simulink model "IEEE9_BUS_with2VSC_VI"  (R2019b)
settings: Solver=ode23tb  StartTime=0.0  StopTime=Tend  RelTol=1e-3
values from neighbouring files (symbols this model uses):
  C_4 = 0.1670*C_b    (= 1.00487241952e-06)    [Basic_Model_Works.m]    (also in VSC_GridFroming_Thesis_Script.m; VSC_GridFroming_Thesis_Script_withSynchMach.m)
  C_6 = 0.2835*C_b    (= 1.70587623314e-06)    [Basic_Model_Works.m]    (also in VSC_GridFroming_Thesis_Script.m; VSC_GridFroming_Thesis_Script_withSynchMach.m)
  C_8 = 0.2275*C_b    (= 1.36891302659e-06)    [Basic_Model_Works.m]    (also in VSC_GridFroming_Thesis_Script.m; VSC_GridFroming_Thesis_Script_withSynchMach.m)
  C_dc = 0.008*(n)    (= 1.6)    [Basic_Model_Works.m]    (also in VSC_GridFroming_Thesis_Script.m; VSC_GridFroming_Thesis_Script_withSynchMach.m)
  C_f = C_f_pu*C1_b    (= 0.0318309886184)    [Basic_Model_Works.m]    (also in VSC_GridFroming_Thesis_Script.m = 0.06; VSC_GridFroming_Thesis_Script_withSynchMach.m)
  droop_percentage = 1    [Basic_Model_Works.m]    (also in VSC_GridFroming_Thesis_Script.m; VSC_GridFroming_Thesis_Script_withSynchMach.m = 5)
  f_b = 50    [Basic_Model_Works.m]    (also in VSC_GridFroming_Thesis_Script.m; VSC_GridFroming_Thesis_Script_withSynchMach.m)
  I_b_LV = S_b/(sqrt(3)*V1_rms)    [Basic_Model_Works.m]    (also in VSC_GridFroming_Thesis_Script.m; VSC_GridFroming_Thesis_Script_withSynchMach.m)
  i_ll = -1.15*(S_b/Vdc_n)-i_loss_dc    [Basic_Model_Works.m]    (also in VSC_GridFroming_Thesis_Script.m; VSC_GridFroming_Thesis_Script_withSynchMach.m)
  I_threshold = I_thresh    (= 1)    [Basic_Model_Works.m]
  i_ul = 1.15*(S_b/Vdc_n)+i_loss_dc    [Basic_Model_Works.m]    (also in VSC_GridFroming_Thesis_Script.m; VSC_GridFroming_Thesis_Script_withSynchMach.m)
  k_dc = eta_1/(Vdc_n*m_p)    [Basic_Model_Works.m]    (also in VSC_GridFroming_Thesis_Script.m; VSC_GridFroming_Thesis_Script_withSynchMach.m)
  K_p = (1/Vdc_n)    [Basic_Model_Works.m]    (also in VSC_GridFroming_Thesis_Script.m; VSC_GridFroming_Thesis_Script_withSynchMach.m)
  K_r = 1/R_dc    [Basic_Model_Works.m]    (also in VSC_GridFroming_Thesis_Script.m; VSC_GridFroming_Thesis_Script_withSynchMach.m)
  Kff_i = 1    [Basic_Model_Works.m]    (also in VSC_GridFroming_Thesis_Script.m; VSC_GridFroming_Thesis_Script_withSynchMach.m)
  Kff_v = 1    [Basic_Model_Works.m]    (also in VSC_GridFroming_Thesis_Script.m; VSC_GridFroming_Thesis_Script_withSynchMach.m)
  Ki_i = (1/n)*1.19    (= 0.00595)    [Basic_Model_Works.m]    (also in VSC_GridFroming_Thesis_Script.m; VSC_GridFroming_Thesis_Script_withSynchMach.m)
  Ki_v = (n)*1.16    (= 232)    [Basic_Model_Works.m]    (also in VSC_GridFroming_Thesis_Script.m = 232.2044; VSC_GridFroming_Thesis_Script_withSynchMach.m = 232.2044)
  ki_v_ac = 10    [Basic_Model_Works.m]    (also in VSC_GridFroming_Thesis_Script.m = 0.5; VSC_GridFroming_Thesis_Script_withSynchMach.m)
  Kp_i = 0.73    [Basic_Model_Works.m]    (also in VSC_GridFroming_Thesis_Script.m = 0.738891; VSC_GridFroming_Thesis_Script_withSynchMach.m = 0.738891)
  Kp_v = 0.52    [Basic_Model_Works.m]    (also in VSC_GridFroming_Thesis_Script.m; VSC_GridFroming_Thesis_Script_withSynchMach.m)
  kp_v_ac = 0.05    [Basic_Model_Works.m]    (also in VSC_GridFroming_Thesis_Script.m = 0.001; VSC_GridFroming_Thesis_Script_withSynchMach.m)
  L1_pu = 1*0.0186/m    (= 0.000186)    [Basic_Model_Works.m]    (also in VSC_GridFroming_Thesis_Script.m; VSC_GridFroming_Thesis_Script_withSynchMach.m)
  L2_mh = 0.08    [Basic_Model_Works.m]    (also in VSC_GridFroming_Thesis_Script_withSynchMach.m)
  L_45 = L_lines(2)    [Basic_Model_Works.m]    (also in VSC_GridFroming_Thesis_Script.m; VSC_GridFroming_Thesis_Script_withSynchMach.m)
  L_56 = L_lines(3)    [Basic_Model_Works.m]    (also in VSC_GridFroming_Thesis_Script.m; VSC_GridFroming_Thesis_Script_withSynchMach.m)
  L_67 = L_lines(5)    [Basic_Model_Works.m]    (also in VSC_GridFroming_Thesis_Script.m; VSC_GridFroming_Thesis_Script_withSynchMach.m)
  L_78 = L_lines(6)    [Basic_Model_Works.m]    (also in VSC_GridFroming_Thesis_Script.m; VSC_GridFroming_Thesis_Script_withSynchMach.m)
  L_89 = L_lines(8)    [Basic_Model_Works.m]    (also in VSC_GridFroming_Thesis_Script.m; VSC_GridFroming_Thesis_Script_withSynchMach.m)
  L_94 = L_lines(9)    [Basic_Model_Works.m]    (also in VSC_GridFroming_Thesis_Script.m; VSC_GridFroming_Thesis_Script_withSynchMach.m)
  L_f = L_f_pu*L1_b    (= 4.77464829276e-06)    [Basic_Model_Works.m]    (also in VSC_GridFroming_Thesis_Script.m = 1e-06; VSC_GridFroming_Thesis_Script_withSynchMach.m)
  L_v = L_v_pu*L1_b    (= 9.54929658551e-06)    [Basic_Model_Works.m]    (also in VSC_GridFroming_Thesis_Script.m; VSC_GridFroming_Thesis_Script_withSynchMach.m = 1.59154943092e-07)
  load_step = S_b*load_change    (= 75000000)    [VSC_GridFroming_Thesis_Script.m]    (also in VSC_GridFroming_Thesis_Script_withSynchMach.m = 50000000)
  m_p = (50*(1.025)-  50*(0.975))/(n*VSC_Pn)    (= 1.25e-08)    [Basic_Model_Works.m]    (also in VSC_GridFroming_Thesis_Script.m = 3.14159265359e-08; VSC_GridFroming_Thesis_Script_withSynchMach.m)
  n = 200    [Basic_Model_Works.m]    (also in VSC_GridFroming_Thesis_Script.m; VSC_GridFroming_Thesis_Script_withSynchMach.m)
  Pn = 210* 1e6    (= 210000000)    [Basic_Model_Works.m]    (also in VSC_GridFroming_Thesis_Script_withSynchMach.m)
  ps = 0.67*Ptot_Load/n_gen    (= 0.5025)    [Basic_Model_Works.m]    (also in VSC_GridFroming_Thesis_Script.m = 0.75; VSC_GridFroming_Thesis_Script_withSynchMach.m = 0.65)
  R1_pu = 1*0.00734/m    (= 7.34e-05)    [Basic_Model_Works.m]    (also in VSC_GridFroming_Thesis_Script.m; VSC_GridFroming_Thesis_Script_withSynchMach.m)
  R2_mh = 0.0027    [Basic_Model_Works.m]    (also in VSC_GridFroming_Thesis_Script_withSynchMach.m)
  R_45 = R_lines(2)    [Basic_Model_Works.m]    (also in VSC_GridFroming_Thesis_Script.m; VSC_GridFroming_Thesis_Script_withSynchMach.m)
  R_56 = R_lines(3)    [Basic_Model_Works.m]    (also in VSC_GridFroming_Thesis_Script.m; VSC_GridFroming_Thesis_Script_withSynchMach.m)
  R_67 = R_lines(5)    [Basic_Model_Works.m]    (also in VSC_GridFroming_Thesis_Script.m; VSC_GridFroming_Thesis_Script_withSynchMach.m)
  R_78 = R_lines(6)    [Basic_Model_Works.m]    (also in VSC_GridFroming_Thesis_Script.m; VSC_GridFroming_Thesis_Script_withSynchMach.m)
  R_89 = R_lines(8)    [Basic_Model_Works.m]    (also in VSC_GridFroming_Thesis_Script.m; VSC_GridFroming_Thesis_Script_withSynchMach.m)
  R_94 = R_lines(9)    [Basic_Model_Works.m]    (also in VSC_GridFroming_Thesis_Script.m; VSC_GridFroming_Thesis_Script_withSynchMach.m)
  R_dc = (Vdc_n/(0.05*(S_b)/Vdc_n))    [Basic_Model_Works.m]    (also in VSC_GridFroming_Thesis_Script.m; VSC_GridFroming_Thesis_Script_withSynchMach.m)
  R_f = R_f_pu*Z1_b    (= 5e-05)    [Basic_Model_Works.m]    (also in VSC_GridFroming_Thesis_Script.m = 5e-06; VSC_GridFroming_Thesis_Script_withSynchMach.m)
  R_v = R_v_pu*Z1_b    (= 0.002)    [Basic_Model_Works.m]    (also in VSC_GridFroming_Thesis_Script.m = 0.001; VSC_GridFroming_Thesis_Script_withSynchMach.m = 1e-05)
  S_b = 100*(10^6)    (= 100000000)    [Basic_Model_Works.m]    (also in VSC_GridFroming_Thesis_Script.m; VSC_GridFroming_Thesis_Script_withSynchMach.m)
  T1sc_off = 13.15    [Basic_Model_Works.m]
  T1sc_on = 13    [Basic_Model_Works.m]
  T3sc_off = 30.15    [Basic_Model_Works.m]
  T3sc_on = 30    [Basic_Model_Works.m]
  T_conn = 13    [Basic_Model_Works.m]
  T_discon = 32    [Basic_Model_Works.m]
  T_en = T_conn-0.5    (= 12.5)    [Basic_Model_Works.m]    (also in VSC_GridFroming_Thesis_Script.m = 19.5; VSC_GridFroming_Thesis_Script_withSynchMach.m = 11.5)
  T_loss = Tend    (= 40)    [VSC_GridFroming_Thesis_Script.m]    (also in VSC_GridFroming_Thesis_Script_withSynchMach.m = 35)
  T_s = 1e-4    (= 0.0001)    [Basic_Model_Works.m]    (also in VSC_GridFroming_Thesis_Script.m; VSC_GridFroming_Thesis_Script_withSynchMach.m)
  tau_dc = 0.05    [Basic_Model_Works.m]    (also in VSC_GridFroming_Thesis_Script.m; VSC_GridFroming_Thesis_Script_withSynchMach.m)
  tau_g = 0.25    [Basic_Model_Works.m]    (also in VSC_GridFroming_Thesis_Script.m = 5; VSC_GridFroming_Thesis_Script_withSynchMach.m = 5)
  Tsc_off = 21.15    [Basic_Model_Works.m]    (also in VSC_GridFroming_Thesis_Script_withSynchMach.m = 20.25)
  Tsc_on = 21    [Basic_Model_Works.m]    (also in VSC_GridFroming_Thesis_Script_withSynchMach.m = 20)
  V = 230*(10^3)    (= 230000)    [Basic_Model_Works.m]    (also in VSC_GridFroming_Thesis_Script.m; VSC_GridFroming_Thesis_Script_withSynchMach.m)
  V1_rms = 1000    [Basic_Model_Works.m]    (also in VSC_GridFroming_Thesis_Script.m; VSC_GridFroming_Thesis_Script_withSynchMach.m)
  V2_rms = 13800    [Basic_Model_Works.m]    (also in VSC_GridFroming_Thesis_Script.m; VSC_GridFroming_Thesis_Script_withSynchMach.m)
  V_m = sqrt(2/3)*V1_rms    [Basic_Model_Works.m]    (also in VSC_GridFroming_Thesis_Script.m; VSC_GridFroming_Thesis_Script_withSynchMach.m)
  Vdc_n = 3*V_m    [Basic_Model_Works.m]    (also in VSC_GridFroming_Thesis_Script.m; VSC_GridFroming_Thesis_Script_withSynchMach.m)
  w_c = w_ref/4.95    (= 63.4665182543)    [Basic_Model_Works.m]    (also in VSC_GridFroming_Thesis_Script_withSynchMach.m)
  w_f = 7.5    [Basic_Model_Works.m]    (also in VSC_GridFroming_Thesis_Script.m = 31.4159265359; VSC_GridFroming_Thesis_Script_withSynchMach.m)
  w_ref = 2*pi*f_b    (= 314.159265359)    [Basic_Model_Works.m]    (also in VSC_GridFroming_Thesis_Script.m; VSC_GridFroming_Thesis_Script_withSynchMach.m)
undefined symbols (not defined in the file or in its folder): D1, Delta, i_dc
libraries: powerlib x112, powerlib_meascontrol x40, cstblocks x5, simulink x4, sps_avr x1
(part 3 of 3)

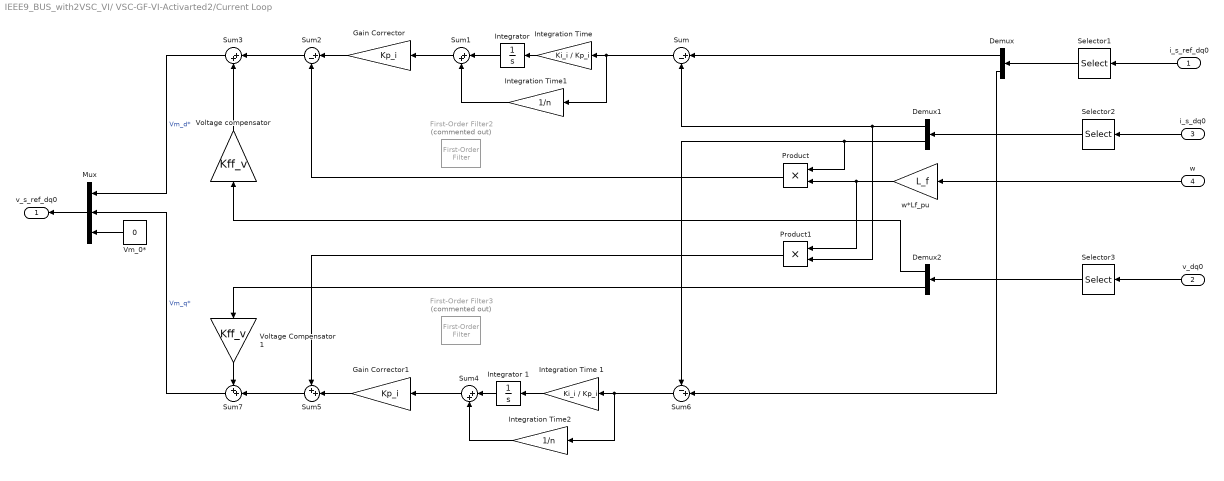
== system IEEE9_BUS_with2VSC_VI/ VSC-GF-VI-Activarted2/Current Loop ==
  i_s_ref_dq0 : Inport
  v_dq0 : Inport  Port=2
  i_s_dq0 : Inport  Port=3
  w : Inport  Port=4
  Demux : Demux  Outputs=2
  Demux1 : Demux  Outputs=2
  Demux2 : Demux  Outputs=2
  First-Order Filter2 : powerlib_meascontrol/Filters/First-Order Filter  Commented=on  FilterType=Lowpass  Tc=25e-3  Ts=0  Initialize=on  Vac_Init=[0, 0, 50]  Vdc_Init=1  PlotResponse=off  FreqRange="[0,  200,  1]"
      settings: SourceProductName=Simscape Electrical
  First-Order Filter3 : powerlib_meascontrol/Filters/First-Order Filter  Commented=on  FilterType=Lowpass  Tc=25e-3  Ts=0  Initialize=on  Vac_Init=[0, 0, 50]  Vdc_Init=0  PlotResponse=off  FreqRange="[0,  200,  1]"
      settings: SourceProductName=Simscape Electrical
  Gain Corrector : Gain  Gain=Kp_i
  Gain Corrector1 : Gain  Gain=Kp_i
  Integration Time : Gain  Gain=Ki_i / Kp_i
  Integration Time 1 : Gain  Gain=Ki_i / Kp_i
  Integration Time1 : Gain  Gain=1/n
  Integration Time2 : Gain  Gain=1/n
  Integrator : Integrator  InitialCondition=0.0001
  Integrator 1 : Integrator
  Mux : Mux  Inputs=3
  Product : Product  RndMeth=Zero
  Product1 : Product  RndMeth=Zero
  Selector1 : Selector  InputPortWidth=3  IndexOptions=Index vector (dialog)  Indices=[1 2]  OutputSizes=1
  Selector2 : Selector  InputPortWidth=3  IndexOptions=Index vector (dialog)  Indices=[1 2]  OutputSizes=1
  Selector3 : Selector  InputPortWidth=3  IndexOptions=Index vector (dialog)  Indices=[1 2]  OutputSizes=1
  Sum : Sum  Inputs=|+-
  Sum1 : Sum  Inputs=|++
  Sum2 : Sum  Inputs=|+-
  Sum3 : Sum  Inputs=|++
  Sum4 : Sum  Inputs=|++
  Sum5 : Sum  Inputs=++|
  Sum6 : Sum  Inputs=-+|
  Sum7 : Sum  Inputs=++|
  Vm_0* : Constant  Value=0
  Voltage Compensator 1 : Gain  Gain=Kff_v
  Voltage compensator : Gain  Gain=Kff_v
  w*Lf_pu : Gain  Gain=L_f
  v_s_ref_dq0 : Outport  VectorParamsAs1DForOutWhenUnconnected=off
  wires:
  Sum/1 -> Integration Time/1, Integration Time1/1
  Integration Time 1/1 -> Integrator 1/1
  Integration Time/1 -> Integrator/1
  Sum5/1 -> Sum7/2
  Sum6/1 -> Integration Time 1/1, Integration Time2/1
  Demux/1 -> Sum/1
  Sum3/1 -> Mux/1  "Vm_d*"
  Sum7/1 -> Mux/2  "Vm_q*"
  Demux2/2 -> Voltage Compensator 1/1
  Voltage Compensator 1/1 -> Sum7/1
  Product/1 -> Sum2/2
  w*Lf_pu/1 -> Product1/1, Product/2
  i_s_ref_dq0/1 -> Selector1/1
  v_dq0/1 -> Selector3/1
  Integrator 1/1 -> Sum4/1
  Voltage compensator/1 -> Sum3/2
  Sum1/1 -> Gain Corrector/1
  Sum2/1 -> Sum3/1
  Sum4/1 -> Gain Corrector1/1
  Demux/2 -> Sum6/2
  Selector1/1 -> Demux/1
  Gain Corrector/1 -> Sum2/1
  w/1 -> w*Lf_pu/1
  Mux/1 -> v_s_ref_dq0/1
  Selector2/1 -> Demux1/1
  i_s_dq0/1 -> Selector2/1
  Selector3/1 -> Demux2/1
  Demux1/2 -> Product/1, Sum6/1
  Vm_0*/1 -> Mux/3
  Integrator/1 -> Sum1/1
  Demux1/1 -> Product1/2, Sum/2
  Demux2/1 -> Voltage compensator/1
  Product1/1 -> Sum5/1
  Gain Corrector1/1 -> Sum5/2
  Integration Time1/1 -> Sum1/2
  Integration Time2/1 -> Sum4/2

== system IEEE9_BUS_with2VSC_VI/ VSC-GF-VI-Activarted2/Droop Control ==
  w_b : Inport
  p_m : Inport  Port=2
  p_set : Inport  Port=3
  v_m : Inport  Port=4
  V_abc : Inport  Port=5
  Demux : Demux  Outputs=3
  Gain20 : Gain  Gain=m_p
  Integrator3 : Integrator
  Mux4 : Mux  Inputs=3
  PID Controller : simulink/Continuous/PID Controller  Controller=PID  Form=Parallel  TimeDomain=Continuous-time  SampleTime=-1  IntegratorMethod=Forward Euler  FilterMethod=Forward Euler  ControllerParametersSource=internal  P=kp_v_ac  I=ki_v_ac  D=0  UseFilter=on  N=100  TunerSelectOption=Transfer Function Based (PID Tuner App)  InitialConditionSource=internal  InitialConditionForIntegrator=0  InitialConditionForFilter=0  DifferentiatorICPrevScaledInput=0  ExternalReset=none  TrackingMode=off  Kt=1  LimitOutput=off  UpperSaturationLimit=inf  LowerSaturationLimit=-inf  LinearizeAsGain=on  AntiWindupMode=none  Kb=1  POutMin=[]  POutMax=[]  IOutMin=[]  IOutMax=[]  DOutMin=[]  DOutMax=[]  NOutMin=[]  NOutMax=[]  SumOutMin=[]  SumOutMax=[]  SaturationOutMin=[]  SaturationOutMax=[]  PParamMin=[]  PParamMax=[]  IParamMin=[]  IParamMax=[]  DParamMin=[]  DParamMax=[]  NParamMin=[]  NParamMax=[]  KbParamMin=[]  KbParamMax=[]  KtParamMin=[]  KtParamMax=[]  KbOutMin=[]  KbOutMax=[]  KtOutMin=[]  KtOutMax=[]  IntegratorOutMin=[]  IntegratorOutMax=[]  FilterOutMin=[]  FilterOutMax=[]  SumI1OutMin=[]  SumI1OutMax=[]  SumI2OutMin=[]  SumI2OutMax=[]  SumI3OutMin=[]  SumI3OutMax=[]  SumI4OutMin=[]  SumI4OutMax=[]  SumDOutMin=[]  SumDOutMax=[]  DifferentiatorOutMin=[]  DifferentiatorOutMax=[]  FilterDiffOutCoefMin=[]  FilterDiffOutCoefMax=[]  ReciprocalOutMin=[]  ReciprocalOutMax=[]  SumDenOutMin=[]  SumDenOutMax=[]  SumNumOutMin=[]  SumNumOutMax=[]  DivideOutMin=[]  DivideOutMax=[]  IntegratorContinuousStateAttributes=''  IntegratorStateMustResolveToSignalObject=off  IntegratorRTWStateStorageClass=Auto  FilterContinuousStateAttributes=''  FilterStateMustResolveToSignalObject=off  FilterRTWStateStorageClass=Auto  ParallelPVariant=InternalParameters  IdealPVariant=Disabled  IVariant=InternalParameters  DVariant=InternalParameters  IntegratorVariant=Continuous  SatVariant=Disabled  AWVariant=Passthrough  PCopyVariant=Disabled  TRVariant=Disabled  FdbkBlocksVariant=Forward  IdealPFdbkVariant=Disabled  SatFdbkVariant=Disabled  DerivativeFilterVariant=ContFilter  NVariant=InternalParameters  NCopyVariant=Disabled  FilterICVariant=InternalICsFilter  IntegratorICVariant=InternalICs  ExternalResetVariant=Disabled  TRSumVariant=Passthrough  SumFdbkVariant=Disabled  SumVariant=Sum_PID
  Sum1 : Sum  Inputs=-+|
  Sum7 : Sum  Inputs=|-+
  Sum8 : Sum  Inputs=++|
  Terminator : Terminator
  Terminator1 : Terminator
  Transfer Fcn1 : TransferFcn  Numerator=[w_f]  Denominator=[1 w_f]
  Transfer Fcn2 : TransferFcn  Numerator=[w_c]  Denominator=[1 w_c]
  abc to dq1 : powerlib_meascontrol/Transformations/abc to dq0  Alignment=90 degrees behind phase A axis
      settings: SourceProductName=Simscape Electrical
  q0 : Constant  Value=0
  w_ref : Outport  VectorParamsAs1DForOutWhenUnconnected=off
  theta_ref : Outport  Port=2  VectorParamsAs1DForOutWhenUnconnected=off
  v_ref_dq0 : Outport  Port=3  VectorParamsAs1DForOutWhenUnconnected=off
  wires:
  q0/1 -> Mux4/3, Mux4/2
  Sum8/1 -> Integrator3/1, w_ref/1
  p_set/1 -> Sum7/2
  w_b/1 -> Sum8/1
  Integrator3/1 -> theta_ref/1
  p_m/1 -> Transfer Fcn1/1
  Sum7/1 -> Gain20/1
  Transfer Fcn1/1 -> Sum7/1
  Gain20/1 -> Transfer Fcn2/1
  Transfer Fcn2/1 -> Sum8/2
  abc to dq1/1 -> Demux/1
  Demux/2 -> Terminator/1
  Demux/3 -> Terminator1/1
  v_m/1 -> Mux4/1
  Mux4/1 -> v_ref_dq0/1

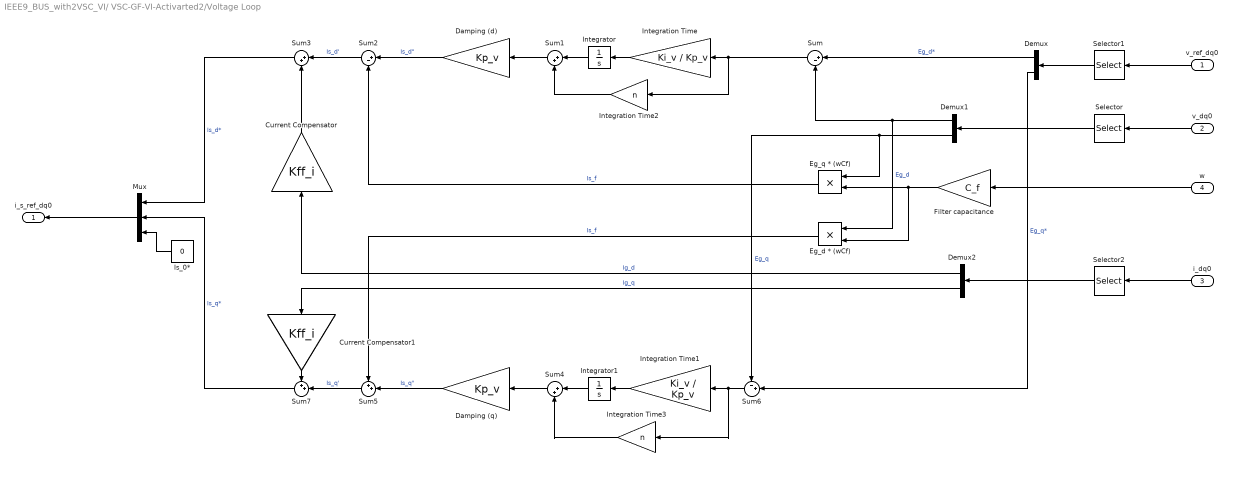
== system IEEE9_BUS_with2VSC_VI/ VSC-GF-VI-Activarted2/Voltage Loop ==
  v_ref_dq0 : Inport
  v_dq0 : Inport  Port=2
  i_dq0 : Inport  Port=3
  w : Inport  Port=4
  Current Compensator : Gain  Gain=Kff_i
  Current Compensator1 : Gain  Gain=Kff_i
  Damping (d) : Gain  Gain=Kp_v
  Damping (q) : Gain  Gain=Kp_v
  Demux : Demux  Outputs=2
  Demux1 : Demux  Outputs=2
  Demux2 : Demux  Outputs=2
  Eg_d * (wCf) : Product  RndMeth=Zero
  "Eg_q * (wCf) " : Product  RndMeth=Zero
  Filter capacitance : Gain  Gain=C_f
  Integration Time : Gain  Gain=Ki_v / Kp_v
  Integration Time1 : Gain  Gain=Ki_v / Kp_v
  Integration Time2 : Gain  Gain=n
  Integration Time3 : Gain  Gain=n
  Integrator : Integrator
  Integrator1 : Integrator
  Is_0* : Constant  Value=0
  Mux : Mux  Inputs=3
  Selector : Selector  InputPortWidth=3  IndexOptions=Index vector (dialog)  Indices=[1 2]  OutputSizes=1
  Selector1 : Selector  InputPortWidth=3  IndexOptions=Index vector (dialog)  Indices=[1 2]  OutputSizes=1
  Selector2 : Selector  InputPortWidth=3  IndexOptions=Index vector (dialog)  Indices=[1 2]  OutputSizes=1
  Sum : Sum  Inputs=|+-
  Sum1 : Sum  Inputs=|++
  Sum2 : Sum  Inputs=|+-
  Sum3 : Sum  Inputs=|++
  Sum4 : Sum  Inputs=|++
  Sum5 : Sum  Inputs=++|
  Sum6 : Sum  Inputs=-+|
  Sum7 : Sum  Inputs=++|
  i_s_ref_dq0 : Outport  VectorParamsAs1DForOutWhenUnconnected=off
  wires:
  Is_0*/1 -> Mux/3
  w/1 -> Filter capacitance/1
  Integration Time1/1 -> Integrator1/1
  Integrator1/1 -> Sum4/1
  Demux/2 -> Sum6/2  "Eg_q*"
  v_ref_dq0/1 -> Selector1/1
  Eg_d * (wCf)/1 -> Sum5/1  "Is_f"
  Sum7/1 -> Mux/2  "Is_q*"
  Demux2/2 -> Current Compensator1/1  "Ig_q"
  Demux/1 -> Sum/1  "Eg_d*"
  Sum6/1 -> Integration Time3/1, Integration Time1/1
  Demux2/1 -> Current Compensator/1  "Ig_d"
  Sum2/1 -> Sum3/1  "Is_d'"
  Current Compensator/1 -> Sum3/2
  Demux1/1 -> Eg_d * (wCf)/1, Sum/2  "Eg_d"
  Current Compensator1/1 -> Sum7/1
  "Eg_q * (wCf) "/1 -> Sum2/2  "Is_f"
  Demux1/2 -> "Eg_q * (wCf) "/1, Sum6/1  "Eg_q"
  Filter capacitance/1 -> "Eg_q * (wCf) "/2, Eg_d * (wCf)/2
  Damping (d)/1 -> Sum2/1  "Is_d\""
  i_dq0/1 -> Selector2/1
  Sum5/1 -> Sum7/2  "Is_q'"
  Sum1/1 -> Damping (d)/1
  Integrator/1 -> Sum1/1
  Integration Time/1 -> Integrator/1
  Sum4/1 -> Damping (q)/1
  Sum3/1 -> Mux/1  "Is_d*"
  v_dq0/1 -> Selector/1
  Damping (q)/1 -> Sum5/2  "Is_q\""
  Selector/1 -> Demux1/1
  Selector1/1 -> Demux/1
  Selector2/1 -> Demux2/1
  Mux/1 -> i_s_ref_dq0/1
  Sum/1 -> Integration Time/1, Integration Time2/1
  Integration Time2/1 -> Sum1/2
  Integration Time3/1 -> Sum4/2

== system IEEE9_BUS_with2VSC_VI/Synchronous Machine/Subsystem2 ==
  P_ref : Inport
  speed_ref : Inport  Port=2
  speed : Inport  Port=3
  1/droop : Gain  Gain=1/((droop_percentage/100))
  Delta load setpoint : Sum  Inputs=+-|
  Delta speed : Sum  Inputs=-+|
  throttle : Outport  VectorParamsAs1DForOutWhenUnconnected=off
  wires:
  speed/1 -> Delta speed/2
  1/droop/1 -> Delta load setpoint/2
  Delta speed/1 -> 1/droop/1
  speed_ref/1 -> Delta speed/1
  P_ref/1 -> Delta load setpoint/1
  Delta load setpoint/1 -> throttle/1

== system IEEE9_BUS_with2VSC_VI/VSC-GF-VI2/ Virtual Impedance ==
  "V_ref_P-w " : Inport
  I_dq0 : Inport  Port=2
  w : Inport  Port=3
  Constant : Constant  Value=0
  Demux4 : Demux  Outputs=2
  "Io_d * (w*Lv) " : Product  RndMeth=Zero
  "Io_q * (w*Lv) " : Product  RndMeth=Zero
  Mux : Mux  Inputs=3
  Selector : Selector  InputPortWidth=3  IndexOptions=Index vector (dialog)  Indices=[1 2]  OutputSizes=1
  Sum : Sum  Inputs=|+-
  Sum4 : Sum  Inputs=|++
  Sum5 : Sum  Inputs=-+|
  Sum6 : Sum  Inputs=-+|
  V_ref_0 : Constant  Value=0
  Virtual indutance : Gain  Gain=L_v
  Virtual resistance : Gain  Gain=R_v
  "Virtual resistance2 " : Gain  Gain=R_v
  V_ref_dq0_VI : Outport
  wires:
  "Io_d * (w*Lv) "/1 -> Sum5/1  "Io_d * (w*Lv)"
  Sum4/1 -> Mux/1
  Virtual indutance/1 -> "Io_q * (w*Lv) "/2, "Io_d * (w*Lv) "/2
  Sum/1 -> Sum4/1
  I_dq0/1 -> Selector/1
  w/1 -> Virtual indutance/1
  Virtual resistance/1 -> Sum/2
  "Virtual resistance2 "/1 -> Sum6/1
  Sum5/1 -> Mux/2
  Selector/1 -> Demux4/1
  Sum6/1 -> Sum5/2
  V_ref_0/1 -> Mux/3
  Demux4/1 -> "Io_d * (w*Lv) "/1, Virtual resistance/1  "Io_d"
  "V_ref_P-w "/1 -> Sum/1  "|v_ref|"
  Constant/1 -> Sum6/2
  "Io_q * (w*Lv) "/1 -> Sum4/2  "Io_q * (w*Lv)"
  Demux4/2 -> "Virtual resistance2 "/1, "Io_q * (w*Lv) "/1  "Io_q"
  Mux/1 -> V_ref_dq0_VI/1

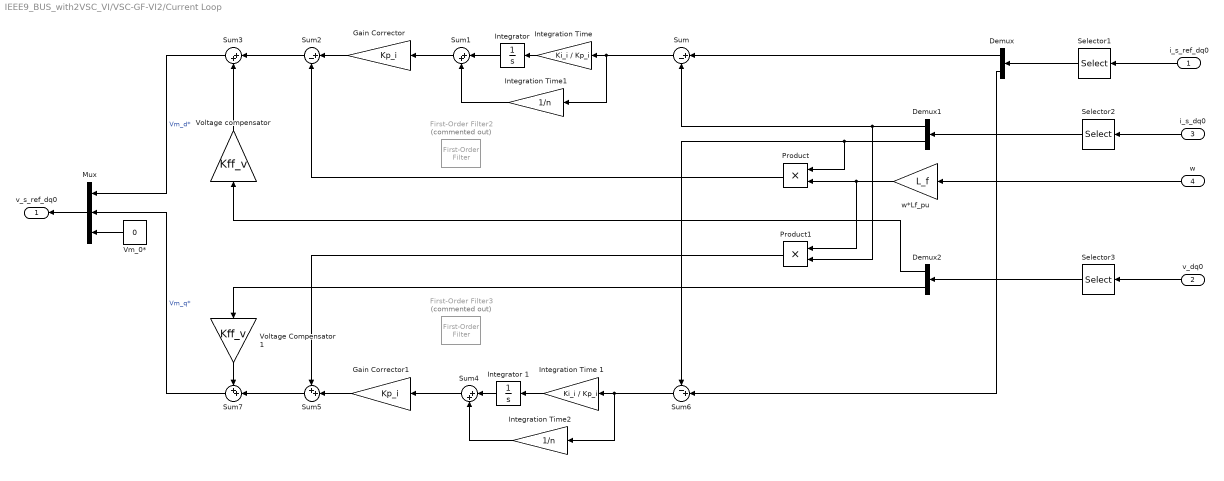
== system IEEE9_BUS_with2VSC_VI/VSC-GF-VI2/Current Loop ==
  i_s_ref_dq0 : Inport
  v_dq0 : Inport  Port=2
  i_s_dq0 : Inport  Port=3
  w : Inport  Port=4
  Demux : Demux  Outputs=2
  Demux1 : Demux  Outputs=2
  Demux2 : Demux  Outputs=2
  First-Order Filter2 : powerlib_meascontrol/Filters/First-Order Filter  Commented=on  FilterType=Lowpass  Tc=25e-3  Ts=0  Initialize=on  Vac_Init=[0, 0, 50]  Vdc_Init=1  PlotResponse=off  FreqRange="[0,  200,  1]"
      settings: SourceProductName=Simscape Electrical
  First-Order Filter3 : powerlib_meascontrol/Filters/First-Order Filter  Commented=on  FilterType=Lowpass  Tc=25e-3  Ts=0  Initialize=on  Vac_Init=[0, 0, 50]  Vdc_Init=0  PlotResponse=off  FreqRange="[0,  200,  1]"
      settings: SourceProductName=Simscape Electrical
  Gain Corrector : Gain  Gain=Kp_i
  Gain Corrector1 : Gain  Gain=Kp_i
  Integration Time : Gain  Gain=Ki_i / Kp_i
  Integration Time 1 : Gain  Gain=Ki_i / Kp_i
  Integration Time1 : Gain  Gain=1/n
  Integration Time2 : Gain  Gain=1/n
  Integrator : Integrator  InitialCondition=0.0001
  Integrator 1 : Integrator
  Mux : Mux  Inputs=3
  Product : Product  RndMeth=Zero
  Product1 : Product  RndMeth=Zero
  Selector1 : Selector  InputPortWidth=3  IndexOptions=Index vector (dialog)  Indices=[1 2]  OutputSizes=1
  Selector2 : Selector  InputPortWidth=3  IndexOptions=Index vector (dialog)  Indices=[1 2]  OutputSizes=1
  Selector3 : Selector  InputPortWidth=3  IndexOptions=Index vector (dialog)  Indices=[1 2]  OutputSizes=1
  Sum : Sum  Inputs=|+-
  Sum1 : Sum  Inputs=|++
  Sum2 : Sum  Inputs=|+-
  Sum3 : Sum  Inputs=|++
  Sum4 : Sum  Inputs=|++
  Sum5 : Sum  Inputs=++|
  Sum6 : Sum  Inputs=-+|
  Sum7 : Sum  Inputs=++|
  Vm_0* : Constant  Value=0
  Voltage Compensator 1 : Gain  Gain=Kff_v
  Voltage compensator : Gain  Gain=Kff_v
  w*Lf_pu : Gain  Gain=L_f
  v_s_ref_dq0 : Outport  VectorParamsAs1DForOutWhenUnconnected=off
  wires:
  Sum/1 -> Integration Time/1, Integration Time1/1
  Integration Time 1/1 -> Integrator 1/1
  Integration Time/1 -> Integrator/1
  Sum5/1 -> Sum7/2
  Sum6/1 -> Integration Time 1/1, Integration Time2/1
  Demux/1 -> Sum/1
  Sum3/1 -> Mux/1  "Vm_d*"
  Sum7/1 -> Mux/2  "Vm_q*"
  Demux2/2 -> Voltage Compensator 1/1
  Voltage Compensator 1/1 -> Sum7/1
  Product/1 -> Sum2/2
  w*Lf_pu/1 -> Product1/1, Product/2
  i_s_ref_dq0/1 -> Selector1/1
  v_dq0/1 -> Selector3/1
  Integrator 1/1 -> Sum4/1
  Voltage compensator/1 -> Sum3/2
  Sum1/1 -> Gain Corrector/1
  Sum2/1 -> Sum3/1
  Sum4/1 -> Gain Corrector1/1
  Demux/2 -> Sum6/2
  Selector1/1 -> Demux/1
  Gain Corrector/1 -> Sum2/1
  w/1 -> w*Lf_pu/1
  Mux/1 -> v_s_ref_dq0/1
  Selector2/1 -> Demux1/1
  i_s_dq0/1 -> Selector2/1
  Selector3/1 -> Demux2/1
  Demux1/2 -> Product/1, Sum6/1
  Vm_0*/1 -> Mux/3
  Integrator/1 -> Sum1/1
  Demux1/1 -> Product1/2, Sum/2
  Demux2/1 -> Voltage compensator/1
  Product1/1 -> Sum5/1
  Gain Corrector1/1 -> Sum5/2
  Integration Time1/1 -> Sum1/2
  Integration Time2/1 -> Sum4/2

== system IEEE9_BUS_with2VSC_VI/VSC-GF-VI2/Droop Control ==
  w_b : Inport
  p_m : Inport  Port=2
  p_set : Inport  Port=3
  v_m : Inport  Port=4
  V_abc : Inport  Port=5
  Demux : Demux  Outputs=3
  Gain20 : Gain  Gain=m_p
  Integrator3 : Integrator
  Mux4 : Mux  Inputs=3
  PID Controller : simulink/Continuous/PID Controller  Controller=PID  Form=Parallel  TimeDomain=Continuous-time  SampleTime=-1  IntegratorMethod=Forward Euler  FilterMethod=Forward Euler  ControllerParametersSource=internal  P=kp_v_ac  I=ki_v_ac  D=0  UseFilter=on  N=100  TunerSelectOption=Transfer Function Based (PID Tuner App)  InitialConditionSource=internal  InitialConditionForIntegrator=0  InitialConditionForFilter=0  DifferentiatorICPrevScaledInput=0  ExternalReset=none  TrackingMode=off  Kt=1  LimitOutput=off  UpperSaturationLimit=inf  LowerSaturationLimit=-inf  LinearizeAsGain=on  AntiWindupMode=none  Kb=1  POutMin=[]  POutMax=[]  IOutMin=[]  IOutMax=[]  DOutMin=[]  DOutMax=[]  NOutMin=[]  NOutMax=[]  SumOutMin=[]  SumOutMax=[]  SaturationOutMin=[]  SaturationOutMax=[]  PParamMin=[]  PParamMax=[]  IParamMin=[]  IParamMax=[]  DParamMin=[]  DParamMax=[]  NParamMin=[]  NParamMax=[]  KbParamMin=[]  KbParamMax=[]  KtParamMin=[]  KtParamMax=[]  KbOutMin=[]  KbOutMax=[]  KtOutMin=[]  KtOutMax=[]  IntegratorOutMin=[]  IntegratorOutMax=[]  FilterOutMin=[]  FilterOutMax=[]  SumI1OutMin=[]  SumI1OutMax=[]  SumI2OutMin=[]  SumI2OutMax=[]  SumI3OutMin=[]  SumI3OutMax=[]  SumI4OutMin=[]  SumI4OutMax=[]  SumDOutMin=[]  SumDOutMax=[]  DifferentiatorOutMin=[]  DifferentiatorOutMax=[]  FilterDiffOutCoefMin=[]  FilterDiffOutCoefMax=[]  ReciprocalOutMin=[]  ReciprocalOutMax=[]  SumDenOutMin=[]  SumDenOutMax=[]  SumNumOutMin=[]  SumNumOutMax=[]  DivideOutMin=[]  DivideOutMax=[]  IntegratorContinuousStateAttributes=''  IntegratorStateMustResolveToSignalObject=off  IntegratorRTWStateStorageClass=Auto  FilterContinuousStateAttributes=''  FilterStateMustResolveToSignalObject=off  FilterRTWStateStorageClass=Auto  ParallelPVariant=InternalParameters  IdealPVariant=Disabled  IVariant=InternalParameters  DVariant=InternalParameters  IntegratorVariant=Continuous  SatVariant=Disabled  AWVariant=Passthrough  PCopyVariant=Disabled  TRVariant=Disabled  FdbkBlocksVariant=Forward  IdealPFdbkVariant=Disabled  SatFdbkVariant=Disabled  DerivativeFilterVariant=ContFilter  NVariant=InternalParameters  NCopyVariant=Disabled  FilterICVariant=InternalICsFilter  IntegratorICVariant=InternalICs  ExternalResetVariant=Disabled  TRSumVariant=Passthrough  SumFdbkVariant=Disabled  SumVariant=Sum_PID
  Sum1 : Sum  Inputs=-+|
  Sum7 : Sum  Inputs=|-+
  Sum8 : Sum  Inputs=++|
  Terminator : Terminator
  Terminator1 : Terminator
  Transfer Fcn1 : TransferFcn  Numerator=[w_f]  Denominator=[1 w_f]
  Transfer Fcn2 : TransferFcn  Numerator=[w_c]  Denominator=[1 w_c]
  abc to dq1 : powerlib_meascontrol/Transformations/abc to dq0  Alignment=90 degrees behind phase A axis
      settings: SourceProductName=Simscape Electrical
  q0 : Constant  Value=0
  w_ref : Outport  VectorParamsAs1DForOutWhenUnconnected=off
  theta_ref : Outport  Port=2  VectorParamsAs1DForOutWhenUnconnected=off
  v_ref_dq0 : Outport  Port=3  VectorParamsAs1DForOutWhenUnconnected=off
  wires:
  q0/1 -> Mux4/3, Mux4/2
  Sum8/1 -> Integrator3/1, w_ref/1
  p_set/1 -> Sum7/2
  w_b/1 -> Sum8/1
  Integrator3/1 -> abc to dq1/2, theta_ref/1
  p_m/1 -> Transfer Fcn1/1
  Sum7/1 -> Gain20/1
  Transfer Fcn1/1 -> Sum7/1
  Gain20/1 -> Transfer Fcn2/1
  Transfer Fcn2/1 -> Sum8/2
  abc to dq1/1 -> Demux/1
  Demux/2 -> Terminator/1
  Demux/3 -> Terminator1/1
  Mux4/1 -> v_ref_dq0/1
  v_m/1 -> Sum1/2
  V_abc/1 -> abc to dq1/1
  Demux/1 -> Sum1/1
  Sum1/1 -> PID Controller/1
  PID Controller/1 -> Mux4/1

== system IEEE9_BUS_with2VSC_VI/VSC-GF-VI2/Voltage Loop ==
  v_ref_dq0 : Inport
  v_dq0 : Inport  Port=2
  i_dq0 : Inport  Port=3
  w : Inport  Port=4
  Current Compensator : Gain  Gain=Kff_i
  Current Compensator1 : Gain  Gain=Kff_i
  Damping (d) : Gain  Gain=Kp_v
  Damping (q) : Gain  Gain=Kp_v
  Demux : Demux  Outputs=2
  Demux1 : Demux  Outputs=2
  Demux2 : Demux  Outputs=2
  Eg_d * (wCf) : Product  RndMeth=Zero
  "Eg_q * (wCf) " : Product  RndMeth=Zero
  Filter capacitance : Gain  Gain=C_f
  Integration Time : Gain  Gain=Ki_v / Kp_v
  Integration Time1 : Gain  Gain=Ki_v / Kp_v
  Integration Time2 : Gain  Gain=n
  Integration Time3 : Gain  Gain=n
  Integrator : Integrator
  Integrator1 : Integrator
  Is_0* : Constant  Value=0
  Mux : Mux  Inputs=3
  Selector : Selector  InputPortWidth=3  IndexOptions=Index vector (dialog)  Indices=[1 2]  OutputSizes=1
  Selector1 : Selector  InputPortWidth=3  IndexOptions=Index vector (dialog)  Indices=[1 2]  OutputSizes=1
  Selector2 : Selector  InputPortWidth=3  IndexOptions=Index vector (dialog)  Indices=[1 2]  OutputSizes=1
  Sum : Sum  Inputs=|+-
  Sum1 : Sum  Inputs=|++
  Sum2 : Sum  Inputs=|+-
  Sum3 : Sum  Inputs=|++
  Sum4 : Sum  Inputs=|++
  Sum5 : Sum  Inputs=++|
  Sum6 : Sum  Inputs=-+|
  Sum7 : Sum  Inputs=++|
  i_s_ref_dq0 : Outport  VectorParamsAs1DForOutWhenUnconnected=off
  wires:
  Is_0*/1 -> Mux/3
  w/1 -> Filter capacitance/1
  Integration Time1/1 -> Integrator1/1
  Integrator1/1 -> Sum4/1
  Demux/2 -> Sum6/2  "Eg_q*"
  v_ref_dq0/1 -> Selector1/1
  Eg_d * (wCf)/1 -> Sum5/1  "Is_f"
  Sum7/1 -> Mux/2  "Is_q*"
  Demux2/2 -> Current Compensator1/1  "Ig_q"
  Demux/1 -> Sum/1  "Eg_d*"
  Sum6/1 -> Integration Time3/1, Integration Time1/1
  Demux2/1 -> Current Compensator/1  "Ig_d"
  Sum2/1 -> Sum3/1  "Is_d'"
  Current Compensator/1 -> Sum3/2
  Demux1/1 -> Eg_d * (wCf)/1, Sum/2  "Eg_d"
  Current Compensator1/1 -> Sum7/1
  "Eg_q * (wCf) "/1 -> Sum2/2  "Is_f"
  Demux1/2 -> "Eg_q * (wCf) "/1, Sum6/1  "Eg_q"
  Filter capacitance/1 -> "Eg_q * (wCf) "/2, Eg_d * (wCf)/2
  Damping (d)/1 -> Sum2/1  "Is_d\""
  i_dq0/1 -> Selector2/1
  Sum5/1 -> Sum7/2  "Is_q'"
  Sum1/1 -> Damping (d)/1
  Integrator/1 -> Sum1/1
  Integration Time/1 -> Integrator/1
  Sum4/1 -> Damping (q)/1
  Sum3/1 -> Mux/1  "Is_d*"
  v_dq0/1 -> Selector/1
  Damping (q)/1 -> Sum5/2  "Is_q\""
  Selector/1 -> Demux1/1
  Selector1/1 -> Demux/1
  Selector2/1 -> Demux2/1
  Mux/1 -> i_s_ref_dq0/1
  Sum/1 -> Integration Time/1, Integration Time2/1
  Integration Time2/1 -> Sum1/2
  Integration Time3/1 -> Sum4/2

== system IEEE9_BUS_with2VSC_VI/VSC-GF-VI3/ Virtual Impedance ==
  "V_ref_P-w " : Inport
  I_dq0 : Inport  Port=2
  w : Inport  Port=3
  Constant : Constant  Value=0
  Demux4 : Demux  Outputs=2
  "Io_d * (w*Lv) " : Product  RndMeth=Zero
  "Io_q * (w*Lv) " : Product  RndMeth=Zero
  Mux : Mux  Inputs=3
  Selector : Selector  InputPortWidth=3  IndexOptions=Index vector (dialog)  Indices=[1 2]  OutputSizes=1
  Sum : Sum  Inputs=|+-
  Sum4 : Sum  Inputs=|++
  Sum5 : Sum  Inputs=-+|
  Sum6 : Sum  Inputs=-+|
  V_ref_0 : Constant  Value=0
  Virtual indutance : Gain  Gain=L_v
  Virtual resistance : Gain  Gain=R_v
  "Virtual resistance2 " : Gain  Gain=R_v
  V_ref_dq0_VI : Outport
  wires:
  "Io_d * (w*Lv) "/1 -> Sum5/1  "Io_d * (w*Lv)"
  Sum4/1 -> Mux/1
  Virtual indutance/1 -> "Io_q * (w*Lv) "/2, "Io_d * (w*Lv) "/2
  Sum/1 -> Sum4/1
  I_dq0/1 -> Selector/1
  w/1 -> Virtual indutance/1
  Virtual resistance/1 -> Sum/2
  "Virtual resistance2 "/1 -> Sum6/1
  Sum5/1 -> Mux/2
  Selector/1 -> Demux4/1
  Sum6/1 -> Sum5/2
  V_ref_0/1 -> Mux/3
  Demux4/1 -> "Io_d * (w*Lv) "/1, Virtual resistance/1  "Io_d"
  "V_ref_P-w "/1 -> Sum/1  "|v_ref|"
  Constant/1 -> Sum6/2
  "Io_q * (w*Lv) "/1 -> Sum4/2  "Io_q * (w*Lv)"
  Demux4/2 -> "Virtual resistance2 "/1, "Io_q * (w*Lv) "/1  "Io_q"
  Mux/1 -> V_ref_dq0_VI/1

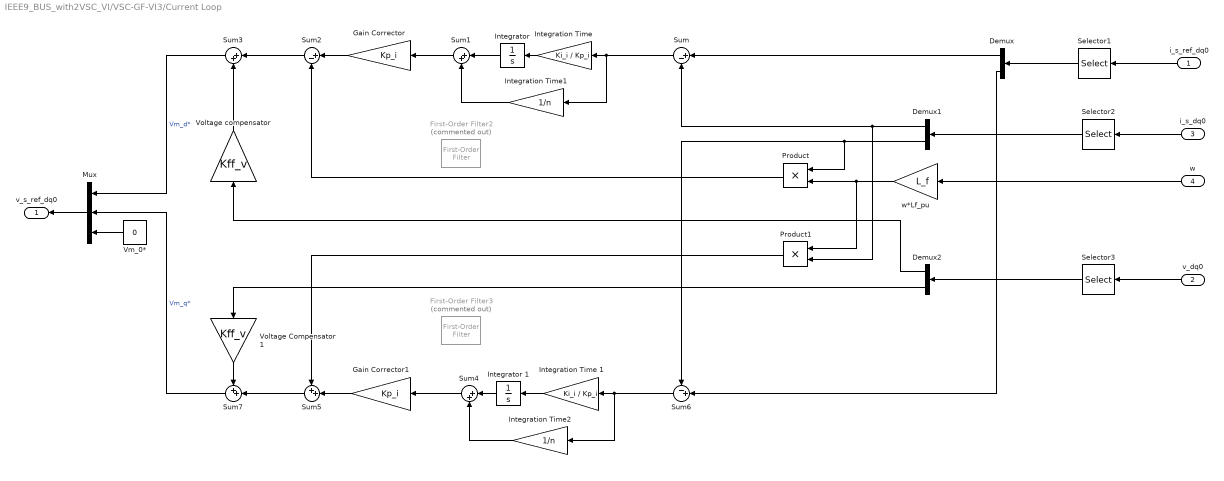
== system IEEE9_BUS_with2VSC_VI/VSC-GF-VI3/Current Loop ==
  i_s_ref_dq0 : Inport
  v_dq0 : Inport  Port=2
  i_s_dq0 : Inport  Port=3
  w : Inport  Port=4
  Demux : Demux  Outputs=2
  Demux1 : Demux  Outputs=2
  Demux2 : Demux  Outputs=2
  First-Order Filter2 : powerlib_meascontrol/Filters/First-Order Filter  Commented=on  FilterType=Lowpass  Tc=25e-3  Ts=0  Initialize=on  Vac_Init=[0, 0, 50]  Vdc_Init=1  PlotResponse=off  FreqRange="[0,  200,  1]"
      settings: SourceProductName=Simscape Electrical
  First-Order Filter3 : powerlib_meascontrol/Filters/First-Order Filter  Commented=on  FilterType=Lowpass  Tc=25e-3  Ts=0  Initialize=on  Vac_Init=[0, 0, 50]  Vdc_Init=0  PlotResponse=off  FreqRange="[0,  200,  1]"
      settings: SourceProductName=Simscape Electrical
  Gain Corrector : Gain  Gain=Kp_i
  Gain Corrector1 : Gain  Gain=Kp_i
  Integration Time : Gain  Gain=Ki_i / Kp_i
  Integration Time 1 : Gain  Gain=Ki_i / Kp_i
  Integration Time1 : Gain  Gain=1/n
  Integration Time2 : Gain  Gain=1/n
  Integrator : Integrator  InitialCondition=0.0001
  Integrator 1 : Integrator
  Mux : Mux  Inputs=3
  Product : Product  RndMeth=Zero
  Product1 : Product  RndMeth=Zero
  Selector1 : Selector  InputPortWidth=3  IndexOptions=Index vector (dialog)  Indices=[1 2]  OutputSizes=1
  Selector2 : Selector  InputPortWidth=3  IndexOptions=Index vector (dialog)  Indices=[1 2]  OutputSizes=1
  Selector3 : Selector  InputPortWidth=3  IndexOptions=Index vector (dialog)  Indices=[1 2]  OutputSizes=1
  Sum : Sum  Inputs=|+-
  Sum1 : Sum  Inputs=|++
  Sum2 : Sum  Inputs=|+-
  Sum3 : Sum  Inputs=|++
  Sum4 : Sum  Inputs=|++
  Sum5 : Sum  Inputs=++|
  Sum6 : Sum  Inputs=-+|
  Sum7 : Sum  Inputs=++|
  Vm_0* : Constant  Value=0
  Voltage Compensator 1 : Gain  Gain=Kff_v
  Voltage compensator : Gain  Gain=Kff_v
  w*Lf_pu : Gain  Gain=L_f
  v_s_ref_dq0 : Outport  VectorParamsAs1DForOutWhenUnconnected=off
  wires:
  Sum/1 -> Integration Time/1, Integration Time1/1
  Integration Time 1/1 -> Integrator 1/1
  Integration Time/1 -> Integrator/1
  Sum5/1 -> Sum7/2
  Sum6/1 -> Integration Time 1/1, Integration Time2/1
  Demux/1 -> Sum/1
  Sum3/1 -> Mux/1  "Vm_d*"
  Sum7/1 -> Mux/2  "Vm_q*"
  Demux2/2 -> Voltage Compensator 1/1
  Voltage Compensator 1/1 -> Sum7/1
  Product/1 -> Sum2/2
  w*Lf_pu/1 -> Product1/1, Product/2
  i_s_ref_dq0/1 -> Selector1/1
  v_dq0/1 -> Selector3/1
  Integrator 1/1 -> Sum4/1
  Voltage compensator/1 -> Sum3/2
  Sum1/1 -> Gain Corrector/1
  Sum2/1 -> Sum3/1
  Sum4/1 -> Gain Corrector1/1
  Demux/2 -> Sum6/2
  Selector1/1 -> Demux/1
  Gain Corrector/1 -> Sum2/1
  w/1 -> w*Lf_pu/1
  Mux/1 -> v_s_ref_dq0/1
  Selector2/1 -> Demux1/1
  i_s_dq0/1 -> Selector2/1
  Selector3/1 -> Demux2/1
  Demux1/2 -> Product/1, Sum6/1
  Vm_0*/1 -> Mux/3
  Integrator/1 -> Sum1/1
  Demux1/1 -> Product1/2, Sum/2
  Demux2/1 -> Voltage compensator/1
  Product1/1 -> Sum5/1
  Gain Corrector1/1 -> Sum5/2
  Integration Time1/1 -> Sum1/2
  Integration Time2/1 -> Sum4/2

== system IEEE9_BUS_with2VSC_VI/VSC-GF-VI3/Droop Control ==
  w_b : Inport
  p_m : Inport  Port=2
  p_set : Inport  Port=3
  v_m : Inport  Port=4
  V_abc : Inport  Port=5
  Demux : Demux  Outputs=3
  Gain20 : Gain  Gain=m_p
  Integrator3 : Integrator
  Mux4 : Mux  Inputs=3
  PID Controller : simulink/Continuous/PID Controller  Controller=PID  Form=Parallel  TimeDomain=Continuous-time  SampleTime=-1  IntegratorMethod=Forward Euler  FilterMethod=Forward Euler  ControllerParametersSource=internal  P=kp_v_ac  I=ki_v_ac  D=0  UseFilter=on  N=100  TunerSelectOption=Transfer Function Based (PID Tuner App)  InitialConditionSource=internal  InitialConditionForIntegrator=0  InitialConditionForFilter=0  DifferentiatorICPrevScaledInput=0  ExternalReset=none  TrackingMode=off  Kt=1  LimitOutput=off  UpperSaturationLimit=inf  LowerSaturationLimit=-inf  LinearizeAsGain=on  AntiWindupMode=none  Kb=1  POutMin=[]  POutMax=[]  IOutMin=[]  IOutMax=[]  DOutMin=[]  DOutMax=[]  NOutMin=[]  NOutMax=[]  SumOutMin=[]  SumOutMax=[]  SaturationOutMin=[]  SaturationOutMax=[]  PParamMin=[]  PParamMax=[]  IParamMin=[]  IParamMax=[]  DParamMin=[]  DParamMax=[]  NParamMin=[]  NParamMax=[]  KbParamMin=[]  KbParamMax=[]  KtParamMin=[]  KtParamMax=[]  KbOutMin=[]  KbOutMax=[]  KtOutMin=[]  KtOutMax=[]  IntegratorOutMin=[]  IntegratorOutMax=[]  FilterOutMin=[]  FilterOutMax=[]  SumI1OutMin=[]  SumI1OutMax=[]  SumI2OutMin=[]  SumI2OutMax=[]  SumI3OutMin=[]  SumI3OutMax=[]  SumI4OutMin=[]  SumI4OutMax=[]  SumDOutMin=[]  SumDOutMax=[]  DifferentiatorOutMin=[]  DifferentiatorOutMax=[]  FilterDiffOutCoefMin=[]  FilterDiffOutCoefMax=[]  ReciprocalOutMin=[]  ReciprocalOutMax=[]  SumDenOutMin=[]  SumDenOutMax=[]  SumNumOutMin=[]  SumNumOutMax=[]  DivideOutMin=[]  DivideOutMax=[]  IntegratorContinuousStateAttributes=''  IntegratorStateMustResolveToSignalObject=off  IntegratorRTWStateStorageClass=Auto  FilterContinuousStateAttributes=''  FilterStateMustResolveToSignalObject=off  FilterRTWStateStorageClass=Auto  ParallelPVariant=InternalParameters  IdealPVariant=Disabled  IVariant=InternalParameters  DVariant=InternalParameters  IntegratorVariant=Continuous  SatVariant=Disabled  AWVariant=Passthrough  PCopyVariant=Disabled  TRVariant=Disabled  FdbkBlocksVariant=Forward  IdealPFdbkVariant=Disabled  SatFdbkVariant=Disabled  DerivativeFilterVariant=ContFilter  NVariant=InternalParameters  NCopyVariant=Disabled  FilterICVariant=InternalICsFilter  IntegratorICVariant=InternalICs  ExternalResetVariant=Disabled  TRSumVariant=Passthrough  SumFdbkVariant=Disabled  SumVariant=Sum_PID
  Sum1 : Sum  Inputs=-+|
  Sum7 : Sum  Inputs=|-+
  Sum8 : Sum  Inputs=++|
  Terminator : Terminator
  Terminator1 : Terminator
  Transfer Fcn1 : TransferFcn  Numerator=[w_f]  Denominator=[1 w_f]
  Transfer Fcn2 : TransferFcn  Numerator=[w_c]  Denominator=[1 w_c]
  abc to dq1 : powerlib_meascontrol/Transformations/abc to dq0  Alignment=90 degrees behind phase A axis
      settings: SourceProductName=Simscape Electrical
  q0 : Constant  Value=0
  w_ref : Outport  VectorParamsAs1DForOutWhenUnconnected=off
  theta_ref : Outport  Port=2  VectorParamsAs1DForOutWhenUnconnected=off
  v_ref_dq0 : Outport  Port=3  VectorParamsAs1DForOutWhenUnconnected=off
  wires:
  q0/1 -> Mux4/3, Mux4/2
  Sum8/1 -> Integrator3/1, w_ref/1
  p_set/1 -> Sum7/2
  w_b/1 -> Sum8/1
  Integrator3/1 -> abc to dq1/2, theta_ref/1
  p_m/1 -> Transfer Fcn1/1
  Sum7/1 -> Gain20/1
  Transfer Fcn1/1 -> Sum7/1
  Gain20/1 -> Transfer Fcn2/1
  Transfer Fcn2/1 -> Sum8/2
  abc to dq1/1 -> Demux/1
  Demux/2 -> Terminator/1
  Demux/3 -> Terminator1/1
  Mux4/1 -> v_ref_dq0/1
  v_m/1 -> Sum1/2
  V_abc/1 -> abc to dq1/1
  Demux/1 -> Sum1/1
  Sum1/1 -> PID Controller/1
  PID Controller/1 -> Mux4/1

== system IEEE9_BUS_with2VSC_VI/VSC-GF-VI3/Voltage Loop ==
  v_ref_dq0 : Inport
  v_dq0 : Inport  Port=2
  i_dq0 : Inport  Port=3
  w : Inport  Port=4
  Current Compensator : Gain  Gain=Kff_i
  Current Compensator1 : Gain  Gain=Kff_i
  Damping (d) : Gain  Gain=Kp_v
  Damping (q) : Gain  Gain=Kp_v
  Demux : Demux  Outputs=2
  Demux1 : Demux  Outputs=2
  Demux2 : Demux  Outputs=2
  Eg_d * (wCf) : Product  RndMeth=Zero
  "Eg_q * (wCf) " : Product  RndMeth=Zero
  Filter capacitance : Gain  Gain=C_f
  Integration Time : Gain  Gain=Ki_v / Kp_v
  Integration Time1 : Gain  Gain=Ki_v / Kp_v
  Integration Time2 : Gain  Gain=n
  Integration Time3 : Gain  Gain=n
  Integrator : Integrator
  Integrator1 : Integrator
  Is_0* : Constant  Value=0
  Mux : Mux  Inputs=3
  Selector : Selector  InputPortWidth=3  IndexOptions=Index vector (dialog)  Indices=[1 2]  OutputSizes=1
  Selector1 : Selector  InputPortWidth=3  IndexOptions=Index vector (dialog)  Indices=[1 2]  OutputSizes=1
  Selector2 : Selector  InputPortWidth=3  IndexOptions=Index vector (dialog)  Indices=[1 2]  OutputSizes=1
  Sum : Sum  Inputs=|+-
  Sum1 : Sum  Inputs=|++
  Sum2 : Sum  Inputs=|+-
  Sum3 : Sum  Inputs=|++
  Sum4 : Sum  Inputs=|++
  Sum5 : Sum  Inputs=++|
  Sum6 : Sum  Inputs=-+|
  Sum7 : Sum  Inputs=++|
  i_s_ref_dq0 : Outport  VectorParamsAs1DForOutWhenUnconnected=off
  wires:
  Is_0*/1 -> Mux/3
  w/1 -> Filter capacitance/1
  Integration Time1/1 -> Integrator1/1
  Integrator1/1 -> Sum4/1
  Demux/2 -> Sum6/2  "Eg_q*"
  v_ref_dq0/1 -> Selector1/1
  Eg_d * (wCf)/1 -> Sum5/1  "Is_f"
  Sum7/1 -> Mux/2  "Is_q*"
  Demux2/2 -> Current Compensator1/1  "Ig_q"
  Demux/1 -> Sum/1  "Eg_d*"
  Sum6/1 -> Integration Time3/1, Integration Time1/1
  Demux2/1 -> Current Compensator/1  "Ig_d"
  Sum2/1 -> Sum3/1  "Is_d'"
  Current Compensator/1 -> Sum3/2
  Demux1/1 -> Eg_d * (wCf)/1, Sum/2  "Eg_d"
  Current Compensator1/1 -> Sum7/1
  "Eg_q * (wCf) "/1 -> Sum2/2  "Is_f"
  Demux1/2 -> "Eg_q * (wCf) "/1, Sum6/1  "Eg_q"
  Filter capacitance/1 -> "Eg_q * (wCf) "/2, Eg_d * (wCf)/2
  Damping (d)/1 -> Sum2/1  "Is_d\""
  i_dq0/1 -> Selector2/1
  Sum5/1 -> Sum7/2  "Is_q'"
  Sum1/1 -> Damping (d)/1
  Integrator/1 -> Sum1/1
  Integration Time/1 -> Integrator/1
  Sum4/1 -> Damping (q)/1
  Sum3/1 -> Mux/1  "Is_d*"
  v_dq0/1 -> Selector/1
  Damping (q)/1 -> Sum5/2  "Is_q\""
  Selector/1 -> Demux1/1
  Selector1/1 -> Demux/1
  Selector2/1 -> Demux2/1
  Mux/1 -> i_s_ref_dq0/1
  Sum/1 -> Integration Time/1, Integration Time2/1
  Integration Time2/1 -> Sum1/2
  Integration Time3/1 -> Sum4/2
